simulink model "pi_sim_2022b"  (R2023b)
settings: Solver=ode45  StartTime=0.0  StopTime=6*60  FixedStep=0.1  RelTol=1e-3  EnableMultiTasking=on
undefined symbols (not defined in the file or in its folder): Advantech, PCI
libraries: sldrtlib x4
settings Model: Creator=Admin  LastModifiedBy=andre
settings SolverCC: AlgebraicLoopSolver=TrustRegion
settings DataIOCC: LimitDataPoints=on  SaveFormat=Array  ReturnWorkspaceOutputs=off
settings OptimizationCC: ReuseModelBlockBuffer=off  LifeSpan=inf
settings DebuggingCC: UnconnectedInputMsg=warning  UnconnectedOutputMsg=warning  UnconnectedLineMsg=warning  SFUnexpectedBacktrackingDiag=warning  SFNoUnconditionalDefaultTransitionDiag=warning  SFExecutionAtInitializationDiag=none  ArithmeticOperatorsInVariantConditions=warning
settings HardwareCC: ProdBitPerPointer=32  ProdBitPerSizeT=32  ProdBitPerPtrDiffT=32  ProdLargestAtomicFloat=None  ProdIntDivRoundTo=Undefined  ProdEndianess=Unspecified  ProdWordSize=32  ProdHWDeviceType=32-bit Generic
settings ModelReferenceCC: PropagateSignalLabelsOutOfModel=off
settings SFSimCC: SimUseLocalCustomCode=off  CustomCodeUndefinedFunction=UseInterfaceOnly
settings RTWCC: RTWUseLocalCustomCode=off
settings CodeAppCC: StateflowObjectComments=on
settings GRTTargetCC: TargetLangStandard=C89/C90 (ANSI)
settings ConfigComp: CovMetricSettings=dw  CovSaveCumulativeToWorkspaceVar=on  CovSaveSingleToWorkspaceVar=on  CovExternalEMLEnable=off

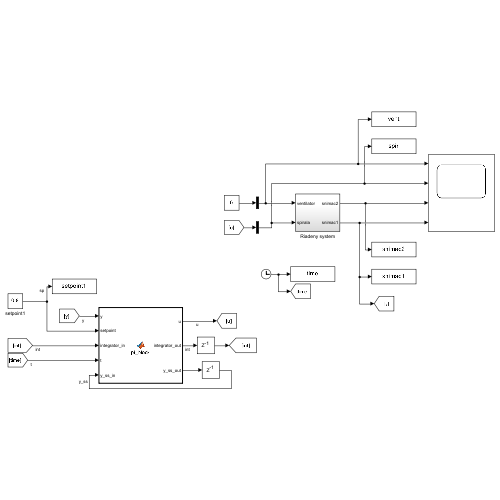
[thumbnail: Simulink's stored preview of the top-level diagram]
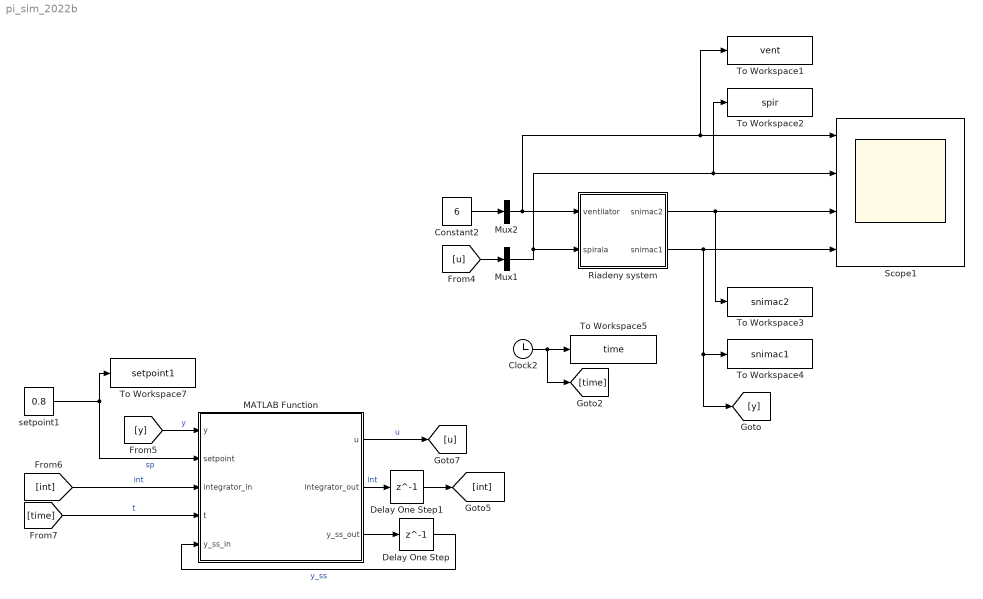
== system pi_sim_2022b ==
  Clock2 : Clock
  Constant2 : Constant  Value=6
  Delay One Step : Delay  DelayLength=1
  Delay One Step1 : Delay  DelayLength=1
  MATLAB Function : MATLAB Function  TreatAsAtomicUnit=on
  Mux1 : Mux  Inputs=1
  Mux2 : Mux  Inputs=1
  Riadeny system : Subsystem
  Scope1 : Scope  NumInputPorts=4
  To Workspace1 : ToWorkspace  VariableName=vent  SampleTime=0.1
      settings: Save2DSignal=2-D array (concatenate along first dimension)
  To Workspace2 : ToWorkspace  VariableName=spir  SampleTime=0.1
      settings: Save2DSignal=2-D array (concatenate along first dimension)
  To Workspace3 : ToWorkspace  VariableName=snimac2  SampleTime=0.1
      settings: Save2DSignal=2-D array (concatenate along first dimension)
  To Workspace4 : ToWorkspace  VariableName=snimac1  SampleTime=0.1
      settings: Save2DSignal=2-D array (concatenate along first dimension)
  To Workspace5 : ToWorkspace  VariableName=time  SampleTime=0.1
      settings: Save2DSignal=2-D array (concatenate along first dimension)
  To Workspace7 : ToWorkspace  VariableName=setpoint1  SampleTime=0.1
      settings: Save2DSignal=2-D array (concatenate along first dimension)
  setpoint1 : Constant  Value=0.8
  wires:
  Delay One Step/1 -> MATLAB Function/5(y_ss_in)  "y_ss"
  [time] -> MATLAB Function/4(t)  "t"
  [int] -> MATLAB Function/3(integrator_in)  "int"
  setpoint1/1 -> To Workspace7/1, MATLAB Function/2(setpoint)  "sp"
  [y] -> MATLAB Function/1(y)  "y"
  MATLAB Function/3(y_ss_out) -> Delay One Step/1
  MATLAB Function/2(integrator_out) -> Delay One Step1/1  "int"
  MATLAB Function/1(u) -> [u]  "u"
  Delay One Step1/1 -> [int]
  [u] -> Mux1/1
  Mux1/1 -> Riadeny system/2(spirala), To Workspace2/1, Scope1/2
  Riadeny system/2(snimac1) -> [y], To Workspace4/1, Scope1/4
  Mux2/1 -> Riadeny system/1(ventilator), To Workspace1/1, Scope1/1
  Riadeny system/1(snimac2) -> To Workspace3/1, Scope1/3
  Clock2/1 -> [time], To Workspace5/1
  Constant2/1 -> Mux2/1

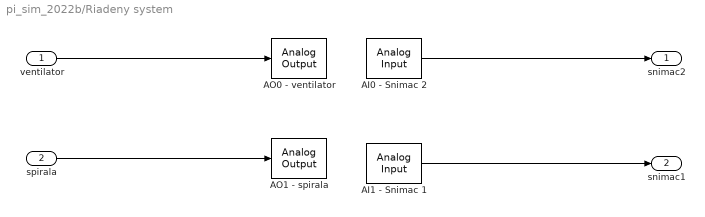
== system pi_sim_2022b/Riadeny system ==
  ventilator : Inport
  spirala : Inport  Port=2
  AI0 - Snimac 2 : sldrtlib/Analog Input  SampleTime=0.1  MaxMissedTicks=10  ShowMissedTicks=off  YieldWhenWaiting=off  DrvName=Advantech/PCI-1711  DrvAddress=4294967295  DrvOptions=zeros(1,0)  Channels=1  RangeMode=1  VoltRange=1  DataType=1
      settings: AttributesFormatString=Advantech\nPCI-1711 [auto]
  AI1 - Snimac 1 : sldrtlib/Analog Input  SampleTime=0.1  MaxMissedTicks=10  ShowMissedTicks=off  YieldWhenWaiting=off  DrvName=Advantech/PCI-1711  DrvAddress=4294967295  DrvOptions=zeros(1,0)  Channels=2  RangeMode=1  VoltRange=1  DataType=1
      settings: AttributesFormatString=Advantech\nPCI-1711 [auto]
  AO0 - ventilator : sldrtlib/Analog Output  SampleTime=0.1  MaxMissedTicks=10  ShowMissedTicks=off  YieldWhenWaiting=off  DrvName=Advantech/PCI-1711  DrvAddress=4294967295  DrvOptions=zeros(1,0)  Channels=1  RangeMode=1  VoltRange=2  InitialValue=[]  FinalValue=[]
      settings: AttributesFormatString=Advantech\nPCI-1711 [auto]
  AO1 - spirala : sldrtlib/Analog Output  SampleTime=0.1  MaxMissedTicks=10  ShowMissedTicks=off  YieldWhenWaiting=off  DrvName=Advantech/PCI-1711  DrvAddress=4294967295  DrvOptions=zeros(1,0)  Channels=2  RangeMode=1  VoltRange=2  InitialValue=[]  FinalValue=[]
      settings: AttributesFormatString=Advantech\nPCI-1711 [auto]
  snimac2 : Outport
  snimac1 : Outport  Port=2
  wires:
  ventilator/1 -> AO0 - ventilator/1
  spirala/1 -> AO1 - spirala/1
  AI1 - Snimac 1/1 -> snimac1/1
  AI0 - Snimac 2/1 -> snimac2/1

== matlab function pi_sim_2022b/MATLAB Function ==
  data: y input; u output; setpoint input; integrator_in input; t input; y_ss_in input; integrator_out output; y_ss_out output
function [u, integrator_out, y_ss_out] = pi_block(y, setpoint, integrator_in, t, y_ss_in)

% PI controller

% Inputs:
%   y            
%   setpoint       
%   integrator_in  
%   Kp, Ki        

% Outputs:
%   u            
%   integrator_out 

    pb_u = 4;
    Ts = 0.1;  
    u_min = - pb_u;
    u_max = 10 - pb_u;
    Kp = 6.76;
    Ki = 2.12;

    %init state of integrator

    if t < 3*60
        u = 4;
        y_ss_out = y;
        integrator_out = 0;
    else
        
        y_ss_out = y_ss_in;
        pb_y = y_ss_in;
        %Outputs normalization
        y = y - pb_y; 

        % PI control law
        e = setpoint - y;

        integrator_out = integrator_in + e * Ts;

        u = Kp * e + Ki * integrator_out;
        u = min(max(u, u_min), u_max);

        %Inputs normalization
        u = u + pb_u;

    end

end
